simulink model "Model_HVAC_old_controller"  (R2019b)
settings: Solver=VariableStepAuto  StartTime=0.0  StopTime=365*24  RelTol=1e-3
undefined symbols (not defined in the file or in its folder): sigbuilder_block, T_s_in
libraries: simulink x1
(part 1 of 2)
settings Model: Creator=HP  LastModifiedBy=HP
settings DebuggingCC: ArithmeticOperatorsInVariantConditions=warning
settings SFSimCC: CustomCodeUndefinedFunction=UseInterfaceOnly

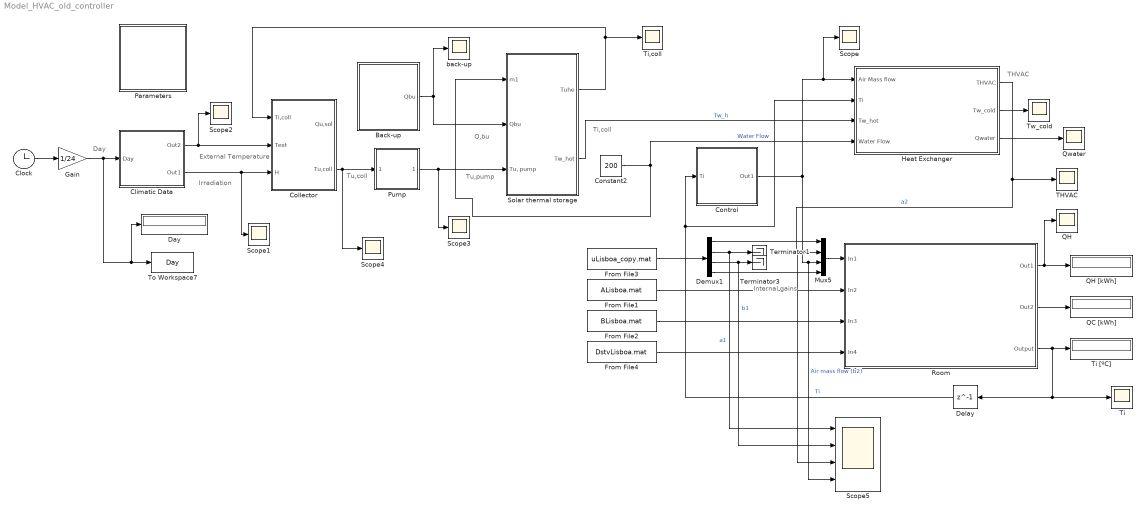
== system Model_HVAC_old_controller ==
  note: THVAC
  note: Internal gains
  note: Tu,pump
  note: Tu,coll
  note: Q,bu
  note: Irradiation
  note: Day
  note: External Temperature
  note: Ti,coll
  Back-up : Subsystem
      mask Display: image(imread('caldaia.jpg'))
  Climatic Data : Subsystem
      mask Display: image(imread('sole.jpg'))
  Clock : Clock
  Collector : Subsystem
      mask Display: image(imread('collettore.jpg'))
  Constant2 : Constant  Value=200
  Control : Subsystem
      mask Display: image('PID.jpg'); % Use "Edit Image" on toolstrip to change.
  Day : Display
  Delay : Delay  DelayLength=1
  Demux1 : Demux  Outputs=[1 1 1 2]
  From File1 : FromFile  FileName=ALisboa.mat  SampleTime=1
  From File2 : FromFile  FileName=BLisboa.mat  SampleTime=1
  From File3 : FromFile  FileName=uLisboa_copy.mat  SampleTime=1
  From File4 : FromFile  FileName=DstvLisboa.mat  SampleTime=1
  Gain : Gain  Gain=1/24  SaturateOnIntegerOverflow=on  OutDataTypeStr=Inherit: Same as input  ParamDataTypeStr=Inherit: Same as input
  Heat Exchanger : Subsystem
      mask Display: image('HE2.jpg'); % Use "Edit Image" on toolstrip to change.
  Mux5 : Mux
  Parameters : Subsystem  mask{Gamma=0, Rho=0.2, Lat=38.74, Beta=45, Eta0=0.959, a1=8.91, a2=0.047, Nc=1, Aap=2.31, m_brine=0.010, Cp_brine=3900, L=1.7, Eta_pump=0.8, Eta_el=0.95, H_pressure=50000, Pump_power=65, Rho_brine=1037, T_room=20, BU_power=2000, Rho_water=1000, Cp_water=4186, U_s=1, T_s_in=45, D_s=0.6, V_s=168, H_s=0.99, UA_s_ex=167, T_s_max=90, A_s_ex=1.8, U_s_ex=1.1, T_DHW=60, S_u=200, T_acq=15}
      mask prompts: Gamma "Azimuth (°)"; Rho "Albedo"; Lat "Latitude (°)"; Beta "Tilt (°)"; Eta0 "Optical efficiency"; a1 "First order coefficient"; a2 "Second order coefficient"; Nc "Number of collectors"; Aap "Absorber area (m2)"; m_brine "Flow rate per surface area (kg/s*m2)"; Cp_brine "Cp brine (J/kgK)"; L "Collector liquid volume (lt)"; Eta_pump "Pump efficiency"; Eta_el "Electrical efficiency"; H_pressure "Head pressure (Pa)"; Pump_power "Pump power (W)"; Rho_brine "Brine density (kg/m3)"; T_room "Room temperature (°C)"; BU_power "Back-up power (W)"; Rho_water "Water density (kg/m3)"; Cp_water "Cp water (J/kgK)"; U_s "Storage U (W/m2K)"; T_s_in "Initial storage temperature (°C)"; D_s "Storage diameter (m)"; V_s "Storage volume (lt)"; H_s "Storage height (m)"; UA_s_ex "Solar exchanger UA (W/K)"; T_s_max "Maximum storage temperature (°C)"; A_s_ex "Heat exchanger area (m2)"; U_s_ex "U-value heat exchanger (W/m2K)"; T_DHW "DHW temperature (°C)"; S_u "Building energetic surface (m2)"; T_acq "Aqueduct temperature (°C)"
      mask Display: image(imread('images.jpg'))
  Pump : Subsystem
      mask Display: image(imread('pompa.jpg'))
  QC [kWh] : Display
      settings: Format=bank  SampleTime=1
  QH : Scope
  QH [kWh] : Display
      settings: Format=bank  SampleTime=1
  Qwater : Scope
  Room : Subsystem
      mask Display: image('roomoffice.jpg'); % Use "Edit Image" on toolstrip to change.
  Scope{,1..4} (5 alike) : Scope
  Scope5 : Scope  NumInputPorts=4
  Solar thermal storage : Subsystem
      mask Display: image(imread('prova.jpg'))
  THVAC : Scope
  Terminator1 : Terminator
  Terminator3 : Terminator
  Ti : Scope
  Ti [ºC] : Display
      settings: Format=bank  SampleTime=1
  Ti,coll : Scope
  To Workspace7 : ToWorkspace  VariableName=Day  SampleTime=[24 0]
  Tw_cold : Scope
  back-up : Scope
  wires:
  Back-up/1(Qbu) -> back-up/1, Solar thermal storage/2(Qbu)
  Solar thermal storage/1(Tuhe) -> Collector/1(Ti,coll), Ti,coll/1
  Gain/1 -> Climatic Data/1(Day), To Workspace7/1, Day/1
  Pump/1(Tu,pump) -> Solar thermal storage/3("Tu, pump"), Scope3/1
  Climatic Data/2(Out1) -> Scope1/1, Collector/3(H)
  Collector/2(Tu,coll) -> Scope4/1, Pump/1(Tu,coll)
  Climatic Data/1(Out2) -> Collector/2(Text), Scope2/1
  Clock/1 -> Gain/1
  Solar thermal storage/2(Tw_hot) -> Heat Exchanger/3(Tw_hot)  "Tw_h"
  Control/1(Out1) -> Scope5/4, Mux5/3, Scope/1, Heat Exchanger/1(Air Mass flow)  "Air mass flow (b2)"
  Heat Exchanger/1(THVAC) -> Scope5/3, Mux5/2, THVAC/1  "a2"
  Heat Exchanger/3(Qwater) -> Qwater/1
  Mux5/1 -> Room/1(In1)
  Heat Exchanger/2(Tw_cold) -> Tw_cold/1
  Delay/1 -> Heat Exchanger/2(Ti), Control/1("Ti ")  "Ti"
  Constant2/1 -> Heat Exchanger/4(Water Flow), Solar thermal storage/1(m1)  "Water Flow"
  Room/3(Output) -> Ti [ºC]/1, Delay/1, Ti/1
  Demux1/3 -> Scope5/2, Terminator3/1  "b1"
  From File4/1 -> Room/4(In4)
  Demux1/2 -> Scope5/1, Terminator1/1  "a1"
  Room/1(Out1) -> QH/1, QH [kWh]/1
  Demux1/4 -> Mux5/4
  From File1/1 -> Room/2(In2)
  From File2/1 -> Room/3(In3)
  Room/2(Out2) -> QC [kWh]/1
  Demux1/1 -> Mux5/1
  From File3/1 -> Demux1/1

== system Model_HVAC_old_controller/Back-up ==
  -Scope : Scope
  -Scope2 : Scope
  Add1 : Sum  Inputs=-+
  Back-up energy [MJ] : Display
  Back-up energy [kWh] : Display
  Constant : Constant  Value=60
  Integral Block : Subsystem
  Product3 : Product  Inputs=**  SaturateOnIntegerOverflow=on  OutDataTypeStr=Inherit: Same as first input
  Prova back-up : Subsystem
  Relay : Relay  OnSwitchValue=0  OffSwitchValue=-5
  Scope : Scope
  To Workspace1 : ToWorkspace  VariableName=Ebu  SampleTime=-1
  To Workspace6 : ToWorkspace  VariableName=Qbu  SampleTime=-1
  Qbu : Outport
  tag scope: Qbu=global
  wires:
  [T3] -> -Scope/1, Add1/1
  Add1/1 -> Relay/1, -Scope2/1
  Relay/1 -> Product3/2
  [BU_power] -> Product3/1
  Product3/1 -> Integral Block/1(Watt), [Qbu], To Workspace6/1, Qbu/1, Scope/1
  Integral Block/1(MJ) -> Back-up energy [MJ]/1
  Integral Block/2(kWh) -> Back-up energy [kWh]/1, To Workspace1/1
  [Tw_hot] -> Add1/2  "Tw_h"
  Constant/1 -> [Tw_hot]

== system Model_HVAC_old_controller/Climatic Data ==
  Day : Inport
  Day Length [h] : Display
  Irradiation : Subsystem  Tag=STV Subsys  LoadFcn=sigbuilder_block('load');  StartFcn=sigbuilder_block('start');  StopFcn=sigbuilder_block('stop');  ClipboardFcn=sigbuilder_block('clipboard');  mask(Sigbuilder block){tuvar=[0:10]}
      mask help: Simulink:masks:SigbuilderBlock_MD
      mask init:
      | if ~strcmp(get_param(bdroot(gcbh),'SimulationStatus'),'stopped') tuvar = sigbuilder_block('maskInit'); end
      settings: CopyFcn=sigbuilder_block('copy');  DeleteFcn=sigbuilder_block('delete');  ModelCloseFcn=sigbuilder_block('modelClose');  PreSaveFcn=sigbuilder_block('preSave');  PauseFcn=sigbuilder_block('pause');  ContinueFcn=sigbuilder_block('continue');  NameChangeFcn=sigbuilder_block('namechange');  OpenFcn=sigbuilder_block('open',[252.75 128.25 550.5 359.25 ]);  CloseFcn=sigbuilder_block('close');
      mask Display: plot(0, 0, 100, 100,[2, 2, 32, 32, 2], [68, 8, 8, 68, 68],[32, 2], [38, 38], [32, 19, 2],[53, 60, 44], [32, 17, 17, 2],[16, 16, 31, 31]);txt = getActiveGroup(gcbh);text(2, 100, txt,'verticalAlignment', 'top');
  Mux4 : Mux  Inputs=2
  Scope : Scope
  Scope1 : Scope
  Scope16 : Scope
  Signal Builder1 : Subsystem  Tag=STV Subsys  LoadFcn=sigbuilder_block('load');  StartFcn=sigbuilder_block('start');  StopFcn=sigbuilder_block('stop');  ClipboardFcn=sigbuilder_block('clipboard');  mask(Sigbuilder block){tuvar=[0:10]}
      mask help: Simulink:masks:SigbuilderBlock_MD
      mask init:
      | if ~strcmp(get_param(bdroot(gcbh),'SimulationStatus'),'stopped') tuvar = sigbuilder_block('maskInit'); end
      settings: CopyFcn=sigbuilder_block('copy');  DeleteFcn=sigbuilder_block('delete');  ModelCloseFcn=sigbuilder_block('modelClose');  PreSaveFcn=sigbuilder_block('preSave');  PauseFcn=sigbuilder_block('pause');  ContinueFcn=sigbuilder_block('continue');  NameChangeFcn=sigbuilder_block('namechange');  OpenFcn=sigbuilder_block('open',[437.6 153 550.4 359.25 ]);  CloseFcn=sigbuilder_block('close');
      mask Display: plot(0, 0, 100, 100,[2, 2, 32, 32, 2], [68, 8, 8, 68, 68],[32, 2], [38, 38], [32, 19, 2],[53, 60, 44], [32, 17, 17, 2],[16, 16, 31, 31]);txt = getActiveGroup(gcbh);text(2, 100, txt,'verticalAlignment', 'top');
  Signal Builder2 : Subsystem  Tag=STV Subsys  LoadFcn=sigbuilder_block('load');  StartFcn=sigbuilder_block('start');  StopFcn=sigbuilder_block('stop');  ClipboardFcn=sigbuilder_block('clipboard');  mask(Sigbuilder block){tuvar=[0:10]}
      mask help: Simulink:masks:SigbuilderBlock_MD
      mask init:
      | if ~strcmp(get_param(bdroot(gcbh),'SimulationStatus'),'stopped') tuvar = sigbuilder_block('maskInit'); end
      settings: CopyFcn=sigbuilder_block('copy');  DeleteFcn=sigbuilder_block('delete');  ModelCloseFcn=sigbuilder_block('modelClose');  PreSaveFcn=sigbuilder_block('preSave');  PauseFcn=sigbuilder_block('pause');  ContinueFcn=sigbuilder_block('continue');  NameChangeFcn=sigbuilder_block('namechange');  OpenFcn=sigbuilder_block('open',[426 129 550.5 359.25 ]);  CloseFcn=sigbuilder_block('close');
      mask Display: plot(0, 0, 100, 100,[2, 2, 32, 32, 2], [68, 8, 8, 68, 68],[32, 2], [38, 38], [32, 19, 2],[53, 60, 44], [32, 17, 17, 2],[16, 16, 31, 31]);txt = getActiveGroup(gcbh);text(2, 100, txt,'verticalAlignment', 'top');
  Signal Builder3 : Subsystem  Tag=STV Subsys  LoadFcn=sigbuilder_block('load');  StartFcn=sigbuilder_block('start');  StopFcn=sigbuilder_block('stop');  ClipboardFcn=sigbuilder_block('clipboard');  mask(Sigbuilder block){tuvar=[0:10]}
      mask help: Simulink:masks:SigbuilderBlock_MD
      mask init:
      | if ~strcmp(get_param(bdroot(gcbh),'SimulationStatus'),'stopped') tuvar = sigbuilder_block('maskInit'); end
      settings: CopyFcn=sigbuilder_block('copy');  DeleteFcn=sigbuilder_block('delete');  ModelCloseFcn=sigbuilder_block('modelClose');  PreSaveFcn=sigbuilder_block('preSave');  PauseFcn=sigbuilder_block('pause');  ContinueFcn=sigbuilder_block('continue');  NameChangeFcn=sigbuilder_block('namechange');  OpenFcn=sigbuilder_block('open',[0 30 1024.5 488.25 ]);  CloseFcn=sigbuilder_block('close');
      mask Display: plot(0, 0, 100, 100,[2, 2, 32, 32, 2], [68, 8, 8, 68, 68],[32, 2], [38, 38], [32, 19, 2],[53, 60, 44], [32, 17, 17, 2],[16, 16, 31, 31]);txt = getActiveGroup(gcbh);text(2, 100, txt,'verticalAlignment', 'top');
  Signal Builder4 : Subsystem  Tag=STV Subsys  LoadFcn=sigbuilder_block('load');  StartFcn=sigbuilder_block('start');  StopFcn=sigbuilder_block('stop');  ClipboardFcn=sigbuilder_block('clipboard');  mask(Sigbuilder block){tuvar=[0:10]}
      mask help: Simulink:masks:SigbuilderBlock_MD
      mask init:
      | if ~strcmp(get_param(bdroot(gcbh),'SimulationStatus'),'stopped') tuvar = sigbuilder_block('maskInit'); end
      settings: CopyFcn=sigbuilder_block('copy');  DeleteFcn=sigbuilder_block('delete');  ModelCloseFcn=sigbuilder_block('modelClose');  PreSaveFcn=sigbuilder_block('preSave');  PauseFcn=sigbuilder_block('pause');  ContinueFcn=sigbuilder_block('continue');  NameChangeFcn=sigbuilder_block('namechange');  OpenFcn=sigbuilder_block('open',[437.6 153 550.4 359.25 ]);  CloseFcn=sigbuilder_block('close');
      mask Display: plot(0, 0, 100, 100,[2, 2, 32, 32, 2], [68, 8, 8, 68, 68],[32, 2], [38, 38], [32, 19, 2],[53, 60, 44], [32, 17, 17, 2],[16, 16, 31, 31]);txt = getActiveGroup(gcbh);text(2, 100, txt,'verticalAlignment', 'top');
  Signal Builder5 : Subsystem  Tag=STV Subsys  LoadFcn=sigbuilder_block('load');  StartFcn=sigbuilder_block('start');  StopFcn=sigbuilder_block('stop');  ClipboardFcn=sigbuilder_block('clipboard');  mask(Sigbuilder block){tuvar=[0:10]}
      mask help: Simulink:masks:SigbuilderBlock_MD
      mask init:
      | if ~strcmp(get_param(bdroot(gcbh),'SimulationStatus'),'stopped') tuvar = sigbuilder_block('maskInit'); end
      settings: CopyFcn=sigbuilder_block('copy');  DeleteFcn=sigbuilder_block('delete');  ModelCloseFcn=sigbuilder_block('modelClose');  PreSaveFcn=sigbuilder_block('preSave');  PauseFcn=sigbuilder_block('pause');  ContinueFcn=sigbuilder_block('continue');  NameChangeFcn=sigbuilder_block('namechange');  OpenFcn=sigbuilder_block('open',[437.6 153 550.4 359.25 ]);  CloseFcn=sigbuilder_block('close');
      mask Display: plot(0, 0, 100, 100,[2, 2, 32, 32, 2], [68, 8, 8, 68, 68],[32, 2], [38, 38], [32, 19, 2],[53, 60, 44], [32, 17, 17, 2],[16, 16, 31, 31]);txt = getActiveGroup(gcbh);text(2, 100, txt,'verticalAlignment', 'top');
  To Workspace2 : ToWorkspace  VariableName=Text  SampleTime=[24 0]
  irraggiamento : Subsystem
  Out2 : Outport  VectorParamsAs1DForOutWhenUnconnected=off
  Out1 : Outport  Port=2  VectorParamsAs1DForOutWhenUnconnected=off
  tag scope: H=global
  wires:
  irraggiamento/1(Out1) -> Day Length [h]/1, Out1/1, Scope/1, [H]
  Mux4/1 -> irraggiamento/1(Climatic Data Input)
  Day/1 -> Mux4/1
  Signal Builder1/1(Temperature) -> Scope16/1, To Workspace2/1, Out2/1
  Irradiation/1(W_45) -> Mux4/2, Scope1/1

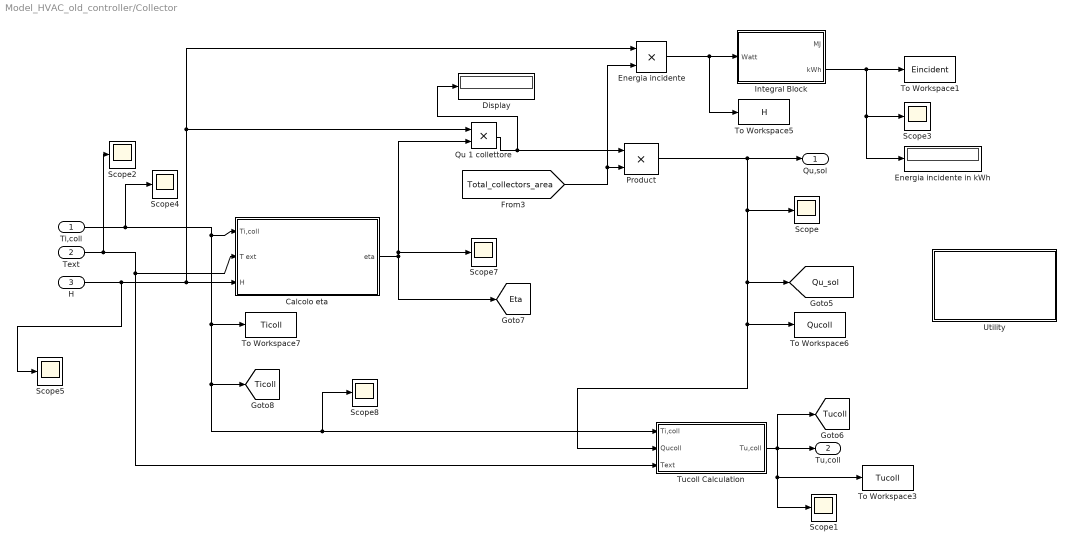
== system Model_HVAC_old_controller/Collector ==
  Ti,coll : Inport
  Text : Inport  Port=2
  H : Inport  Port=3
  Calcolo eta : Subsystem
  Display : Display
  Energia incidente : Product  RndMeth=Zero
  Energia incidente in kWh : Display
  Integral Block : Subsystem
  Product : Product  RndMeth=Zero
  Qu 1 collettore : Product  RndMeth=Zero
  Scope{,1..5,7..8} (8 alike) : Scope
  To Workspace1 : ToWorkspace  VariableName=Eincident  SampleTime=[24 0]
  To Workspace3 : ToWorkspace  VariableName=Tucoll  SampleTime=[24 0]
  To Workspace5 : ToWorkspace  VariableName=H  SampleTime=-1
  To Workspace6 : ToWorkspace  VariableName=Qucoll  SampleTime=[24 0]
  To Workspace7 : ToWorkspace  VariableName=Ticoll  SampleTime=[24 0]
  Tucoll Calculation : Subsystem
  Utility : Subsystem
  Qu,sol : Outport  VectorParamsAs1DForOutWhenUnconnected=off
  Tu,coll : Outport  Port=2  VectorParamsAs1DForOutWhenUnconnected=off
  tag scope: Eta=global, Qu_sol=global, Ticoll=global, Tucoll=global
  wires:
  H/1 -> Scope5/1, Calcolo eta/3(H), Qu 1 collettore/1, Energia incidente/1
  Text/1 -> Scope2/1, Calcolo eta/2(T ext), Tucoll Calculation/3(Text)
  Calcolo eta/1(eta) -> Qu 1 collettore/2, Scope7/1, [Eta]
  Qu 1 collettore/1 -> Product/1, Display/1
  Tucoll Calculation/1(Tu,coll) -> Tu,coll/1, Scope1/1, To Workspace3/1, [Tucoll]
  Energia incidente/1 -> Integral Block/1(Watt), To Workspace5/1
  Product/1 -> Qu,sol/1, [Qu_sol], To Workspace6/1, Tucoll Calculation/2(Qucoll), Scope/1
  Ti,coll/1 -> Scope4/1, [Ticoll], Tucoll Calculation/1(Ti,coll), Scope8/1, To Workspace7/1, Calcolo eta/1(Ti,coll)
  Integral Block/2(kWh) -> To Workspace1/1, Scope3/1, Energia incidente in kWh/1
  [Total_collectors_area] -> Product/2, Energia incidente/2

== system Model_HVAC_old_controller/Control ==
  "Ti " : Inport
  Constant : Constant  Value=24
  Discrete PID Controller (2DOF)1 : simulink/Continuous/PID Controller (2DOF)  Controller=PID  Form=Parallel  TimeDomain=Discrete-time  SampleTime=-1  IntegratorMethod=Forward Euler  FilterMethod=Forward Euler  ControllerParametersSource=internal  P=500  I=100  D=0  UseFilter=on  N=100  b=1  c=1  TunerSelectOption=Transfer Function Based (PID Tuner App)  InitialConditionSource=internal  InitialConditionForIntegrator=0  InitialConditionForFilter=0  DifferentiatorICPrevScaledInput=0  ExternalReset=none  TrackingMode=off  Kt=1  LimitOutput=off  UpperSaturationLimit=inf  LowerSaturationLimit=-inf  LinearizeAsGain=off  AntiWindupMode=none  Kb=1  POutMin=[]  POutMax=[]  IOutMin=[]  IOutMax=[]  DOutMin=[]  DOutMax=[]  NOutMin=[]  NOutMax=[]  bOutMin=[]  bOutMax=[]  cOutMin=[]  cOutMax=[]  SumOutMin=[]  SumOutMax=[]  SaturationOutMin=[]  SaturationOutMax=[]  PParamMin=[]  PParamMax=[]  IParamMin=[]  IParamMax=[]  DParamMin=[]  DParamMax=[]  NParamMin=[]  NParamMax=[]  bParamMin=[]  bParamMax=[]  cParamMin=[]  cParamMax=[]  KbParamMin=[]  KbParamMax=[]  KtParamMin=[]  KtParamMax=[]  KbOutMin=[]  KbOutMax=[]  KtOutMin=[]  KtOutMax=[]  IntegratorOutMin=[]  IntegratorOutMax=[]  FilterOutMin=[]  FilterOutMax=[]  SumI1OutMin=[]  SumI1OutMax=[]  SumI2OutMin=[]  SumI2OutMax=[]  SumI3OutMin=[]  SumI3OutMax=[]  SumI4OutMin=[]  SumI4OutMax=[]  SumDOutMin=[]  SumDOutMax=[]  Sum1OutMin=[]  Sum1OutMax=[]  Sum2OutMin=[]  Sum2OutMax=[]  Sum3OutMin=[]  Sum3OutMax=[]  DifferentiatorOutMin=[]  DifferentiatorOutMax=[]  FilterDiffOutCoefMin=[]  FilterDiffOutCoefMax=[]  ReciprocalOutMin=[]  ReciprocalOutMax=[]  SumDenOutMin=[]  SumDenOutMax=[]  SumNumOutMin=[]  SumNumOutMax=[]  DivideOutMin=[]  DivideOutMax=[]  IntegratorContinuousStateAttributes=''  IntegratorStateMustResolveToSignalObject=off  IntegratorRTWStateStorageClass=Auto  FilterContinuousStateAttributes=''  FilterStateMustResolveToSignalObject=off  FilterRTWStateStorageClass=Auto  ParallelPVariant=InternalParameters  IdealPVariant=Disabled  IVariant=InternalParameters  DVariant=InternalParameters  bVariant=InternalParameters  cVariant=InternalParameters  IntegratorVariant=Discrete  SatVariant=Disabled  AWVariant=Passthrough  PCopyVariant=Disabled  TRVariant=Disabled  FdbkBlocksVariant=Forward  IdealPFdbkVariant=Disabled  SatFdbkVariant=Disabled  DerivativeFilterVariant=ForwardEulerFilter  NVariant=InternalParameters  NCopyVariant=Disabled  FilterICVariant=InternalICsFilter  IntegratorICVariant=InternalICs  ExternalResetVariant=Disabled  TRSumVariant=Passthrough  SumFdbkVariant=Disabled  SumVariant=Sum_PID
  Saturation : Saturate  UpperLimit=1000  LowerLimit=0
  Scope3 : Scope
  Out1 : Outport
  wires:
  Saturation/1 -> Out1/1, Scope3/1  "Air mass flow"
  Discrete PID Controller (2DOF)1/1 -> Saturation/1  "Air mass flow"
  Constant/1 -> Discrete PID Controller (2DOF)1/1
  "Ti "/1 -> Discrete PID Controller (2DOF)1/2

== system Model_HVAC_old_controller/Heat Exchanger ==
  Air Mass flow : Inport
  Ti : Inport  Port=2
  Tw_hot : Inport  Port=3
  Water Flow : Inport  Port=4
  Add : Sum
  Add1 : Sum  Inputs=+-
  Add2 : Sum  Inputs=+-
  Cpair : Constant  Value=1.007
  Cpwater : Constant  Value=4.17
  Divide : Product  Inputs=/**
  Divide1 : Product  Inputs=***
  Divide3 : Product  Inputs=/**
  efficiency : Constant  Value=0.7
  THVAC : Outport
  Tw_cold : Outport  Port=2
  Qwater : Outport  Port=3
  wires:
  Cpair/1 -> Divide1/3, Divide/3
  Air Mass flow/1 -> Divide/2
  Divide/1 -> Add/1
  Ti/1 -> Add/2, Add1/2
  Add/1 -> THVAC/1
  efficiency/1 -> Divide1/2
  Tw_hot/1 -> Add2/1, Add1/1
  Add1/1 -> Divide1/1
  Divide1/1 -> Qwater/1, Divide3/1, Divide/1
  Water Flow/1 -> Divide3/2
  Cpwater/1 -> Divide3/3
  Divide3/1 -> Add2/2
  Add2/1 -> Tw_cold/1

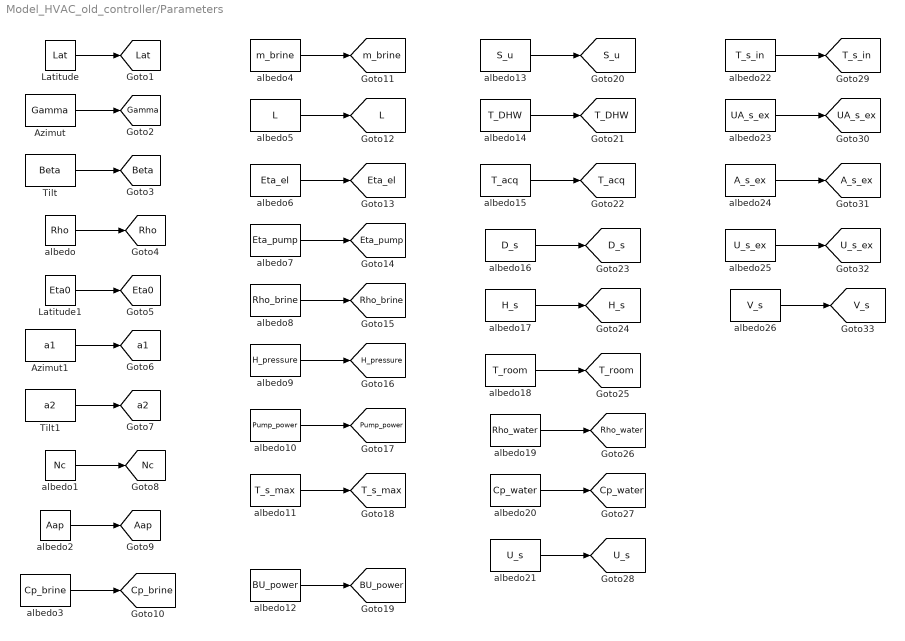
== system Model_HVAC_old_controller/Parameters ==
  Azimut : Constant  Value=Gamma
  Azimut1 : Constant  Value=a1
  Latitude : Constant  Value=Lat
  Latitude1 : Constant  Value=Eta0
  Tilt : Constant  Value=Beta
  Tilt1 : Constant  Value=a2
  albedo : Constant  Value=Rho
  albedo1 : Constant  Value=Nc
  albedo10 : Constant  Value=Pump_power
  albedo11 : Constant  Value=T_s_max
  albedo12 : Constant  Value=BU_power
  albedo13 : Constant  Value=S_u
  albedo14 : Constant  Value=T_DHW
  albedo15 : Constant  Value=T_acq
  albedo16 : Constant  Value=D_s
  albedo17 : Constant  Value=H_s
  albedo18 : Constant  Value=T_room
  albedo19 : Constant  Value=Rho_water
  albedo2 : Constant  Value=Aap
  albedo20 : Constant  Value=Cp_water
  albedo21 : Constant  Value=U_s
  albedo22 : Constant  Value=T_s_in
  albedo23 : Constant  Value=UA_s_ex
  albedo24 : Constant  Value=A_s_ex
  albedo25 : Constant  Value=U_s_ex
  albedo26 : Constant  Value=V_s
  albedo3 : Constant  Value=Cp_brine
  albedo4 : Constant  Value=m_brine
  albedo5 : Constant  Value=L
  albedo6 : Constant  Value=Eta_el
  albedo7 : Constant  Value=Eta_pump
  albedo8 : Constant  Value=Rho_brine
  albedo9 : Constant  Value=H_pressure
  tag scope: A_s_ex=global, Aap=global, BU_power=global, Beta=global, Cp_brine=global, Cp_water=global, D_s=global, Eta0=global, Eta_el=global, Eta_pump=global, Gamma=global, H_pressure=global, H_s=global, L=global, Lat=global, Nc=global, Pump_power=global, Rho=global, Rho_brine=global, Rho_water=global, S_u=global, T_DHW=global, T_acq=global, T_room=global, T_s_in=global, T_s_max=global, UA_s_ex=global, U_s=global, U_s_ex=global, V_s=global, a1=global, a2=global, m_brine=global
  wires:
  Latitude/1 -> [Lat]
  Azimut/1 -> [Gamma]
  Tilt/1 -> [Beta]
  albedo/1 -> [Rho]
  Latitude1/1 -> [Eta0]
  Azimut1/1 -> [a1]
  Tilt1/1 -> [a2]
  albedo1/1 -> [Nc]
  albedo2/1 -> [Aap]
  albedo3/1 -> [Cp_brine]
  albedo4/1 -> [m_brine]
  albedo5/1 -> [L]
  albedo6/1 -> [Eta_el]
  albedo7/1 -> [Eta_pump]
  albedo8/1 -> [Rho_brine]
  albedo9/1 -> [H_pressure]
  albedo10/1 -> [Pump_power]
  albedo11/1 -> [T_s_max]
  albedo12/1 -> [BU_power]
  albedo13/1 -> [S_u]
  albedo14/1 -> [T_DHW]
  albedo15/1 -> [T_acq]
  albedo16/1 -> [D_s]
  albedo17/1 -> [H_s]
  albedo18/1 -> [T_room]
  albedo19/1 -> [Rho_water]
  albedo20/1 -> [Cp_water]
  albedo21/1 -> [U_s]
  albedo22/1 -> [T_s_in]
  albedo23/1 -> [UA_s_ex]
  albedo24/1 -> [A_s_ex]
  albedo25/1 -> [U_s_ex]
  albedo26/1 -> [V_s]

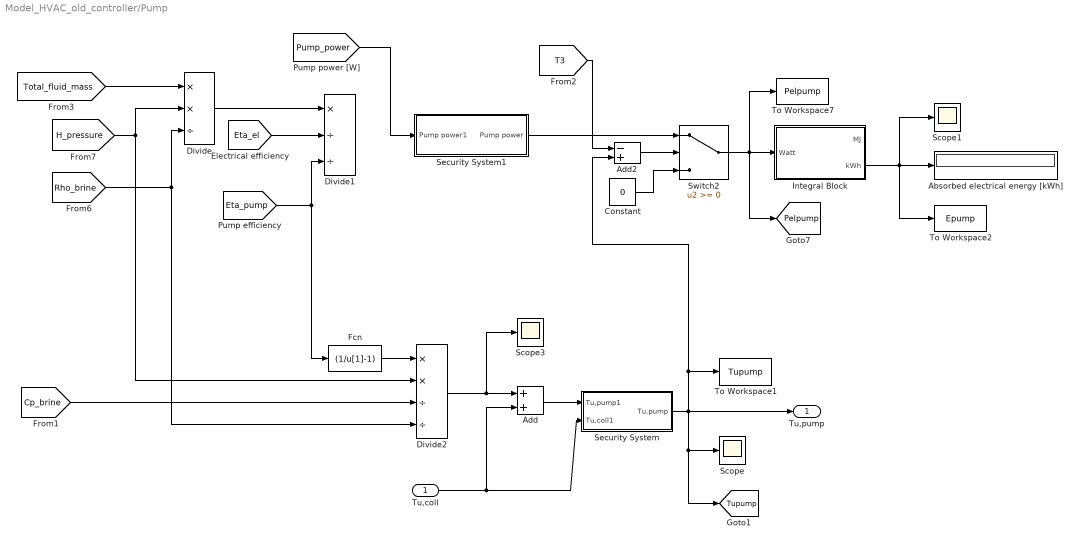
== system Model_HVAC_old_controller/Pump ==
  Tu,coll : Inport
  Absorbed electrical energy [kWh] : Display
  Add : Sum
  Add2 : Sum  Inputs=-+
  Constant : Constant  Value=0
  Divide : Product  Inputs=**/
  Divide1 : Product  Inputs=*//
  Divide2 : Product  Inputs=**//
  Fcn : Fcn  Expr=(1/u[1]-1)
  Integral Block : Subsystem
  Scope : Scope
  Scope1 : Scope
  Scope3 : Scope
  Security System : Subsystem
  Security System1 : Subsystem
  Switch2 : Switch  ZeroCross=off
  To Workspace1 : ToWorkspace  VariableName=Tupump  SampleTime=[24 0]
  To Workspace2 : ToWorkspace  VariableName=Epump  SampleTime=[24 0]
  To Workspace7 : ToWorkspace  VariableName=Pelpump  SampleTime=[24 0]
  Tu,pump : Outport  VectorParamsAs1DForOutWhenUnconnected=off
  tag scope: Pelpump=global, Tupump=global
  wires:
  [Total_fluid_mass] -> Divide/1
  [H_pressure] -> Divide/2, Divide2/2
  [Rho_brine] -> Divide/3, Divide2/4
  Divide/1 -> Divide1/1
  [Eta_pump] -> Fcn/1, Divide1/3
  Fcn/1 -> Divide2/1
  Divide2/1 -> Add/1, Scope3/1
  Tu,coll/1 -> Security System/2(Tu,coll1), Add/2
  [Cp_brine] -> Divide2/3
  Integral Block/2(kWh) -> Absorbed electrical energy [kWh]/1, Scope1/1, To Workspace2/1
  Add/1 -> Security System/1(Tu,pump1)
  Security System/1(Tu,pump) -> To Workspace1/1, Add2/2, Scope/1, [Tupump], Tu,pump/1
  [Eta_el] -> Divide1/2
  [Pump_power] -> Security System1/1(Pump power1)
  Security System1/1(Pump power) -> Switch2/1
  Add2/1 -> Switch2/2
  [T3] -> Add2/1
  Switch2/1 -> To Workspace7/1, [Pelpump], Integral Block/1(Watt)
  Constant/1 -> Switch2/3

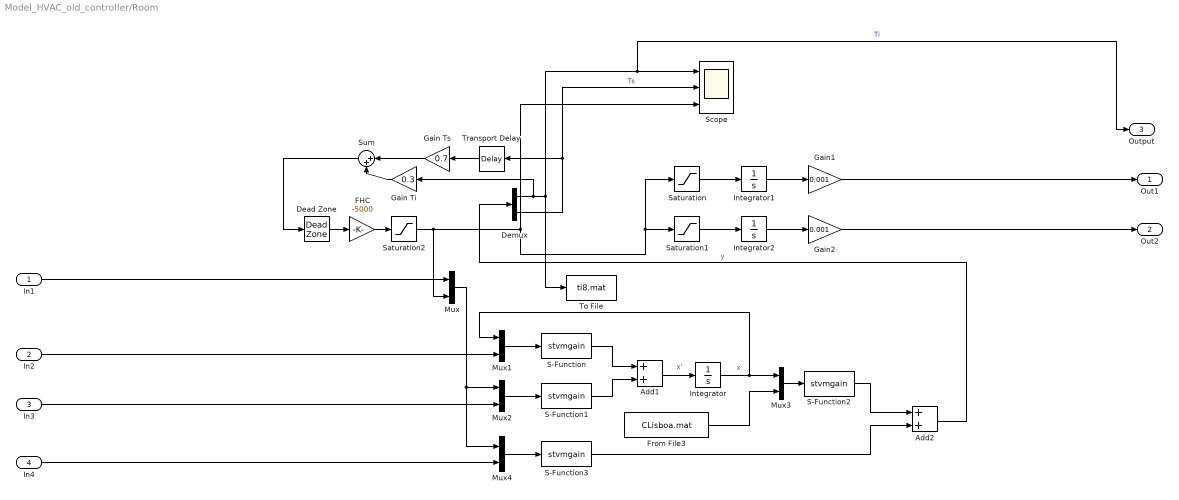
== system Model_HVAC_old_controller/Room ==
  note: x'
  note: x
  In1 : Inport
  In2 : Inport  Port=2
  In3 : Inport  Port=3
  In4 : Inport  Port=4
  Add1 : Sum
  Add2 : Sum
  Dead Zone : DeadZone  LowerValue=20  UpperValue=26  ZeroCross=off  SaturateOnIntegerOverflow=on
  Demux : Demux  Outputs=2
  FHC : Gain  Gain=-5000
  From File3 : FromFile  FileName=CLisboa.mat  SampleTime=1
  Gain Ti : Gain  Gain=0.3
  Gain Ts : Gain  Gain=0.7
  Gain1 : Gain  Gain=0.001  SampleTime=1
  Gain2 : Gain  Gain=0.001  SampleTime=1
  Integrator : Integrator  InitialCondition=18
  Integrator1 : Integrator
  Integrator2 : Integrator
  Mux : Mux  Inputs=2
  Mux1 : Mux  Inputs=[1 1]
  Mux2 : Mux  Inputs=[6 6]
  Mux3 : Mux  Inputs=[1 2]
  Mux4 : Mux  Inputs=[6 12]
  S-Function : S-Function  FunctionName=stvmgain  Parameters=1, -1  SFunctionDeploymentMode=off  EnableBusSupport=off
  S-Function1 : S-Function  FunctionName=stvmgain  Parameters=[1 1 1 1 1 1], -1  SFunctionDeploymentMode=off  EnableBusSupport=off
  S-Function2 : S-Function  FunctionName=stvmgain  Parameters=[1 ;1] -1  SFunctionDeploymentMode=off  EnableBusSupport=off
  S-Function3 : S-Function  FunctionName=stvmgain  Parameters=[1 1 1 1 1 1; 1 1 1 1 1 1], -1  SFunctionDeploymentMode=off  EnableBusSupport=off
  Saturation : Saturate  UpperLimit=20000  LowerLimit=0  SampleTime=1
  Saturation1 : Saturate  UpperLimit=0  LowerLimit=-20000  SampleTime=1
  Saturation2 : Saturate  UpperLimit=10000  LowerLimit=-10000
  Scope : Scope  NumInputPorts=3
  Sum : Sum  Inputs=|++
  To File : ToFile  Filename=ti8.mat  SampleTime=1
  Transport Delay : TransportDelay
  Out1 : Outport  VectorParamsAs1DForOutWhenUnconnected=off
  Out2 : Outport  Port=2  VectorParamsAs1DForOutWhenUnconnected=off
  Output : Outport  Port=3  VectorParamsAs1DForOutWhenUnconnected=off
  wires:
  Sum/1 -> Dead Zone/1
  Mux3/1 -> S-Function2/1
  Demux/1 -> Gain Ti/1, Output/1, Scope/1, To File/1  "Ti"
  Mux2/1 -> S-Function1/1
  Saturation2/1 -> Mux/2, Scope/3, Saturation1/1, Saturation/1
  Mux/1 -> Mux2/1, Mux4/1
  Saturation/1 -> Integrator1/1
  Gain1/1 -> Out1/1
  S-Function/1 -> Add1/1
  Mux4/1 -> S-Function3/1
  Integrator/1 -> Mux3/1, Mux1/1
  FHC/1 -> Saturation2/1
  Saturation1/1 -> Integrator2/1
  Gain Ts/1 -> Sum/1
  Mux1/1 -> S-Function/1
  S-Function3/1 -> Add2/2
  Transport Delay/1 -> Gain Ts/1
  Dead Zone/1 -> FHC/1
  Gain Ti/1 -> Sum/2
  S-Function1/1 -> Add1/2
  Integrator2/1 -> Gain2/1
  Demux/2 -> Scope/2, Transport Delay/1  "Ts"
  In3/1 -> Mux2/2
  Add1/1 -> Integrator/1
  Gain2/1 -> Out2/1
  From File3/1 -> Mux3/2
  In2/1 -> Mux1/2
  S-Function2/1 -> Add2/1
  Integrator1/1 -> Gain1/1
  Add2/1 -> Demux/1  "y"
  In4/1 -> Mux4/2
  In1/1 -> Mux/1

== system Model_HVAC_old_controller/Solar thermal storage ==
  note: V[m3]
  m1 : Inport
  Qbu : Inport  Port=2
  "Tu, pump" : Inport  Port=3
  -Scope1 : Scope
  Divide : Product  Inputs=*/
  Lower part 3 : Subsystem
  Rho water : Constant  Value=1000
  Scope : Scope
  Scope2 : Scope
  Tuhe : Outport  VectorParamsAs1DForOutWhenUnconnected=off
  Tw_hot : Outport  Port=2
  tag scope: m=global
  wires:
  Divide/1 -> Scope2/1, Lower part 3/1(V)
  Rho water/1 -> Divide/2
  Lower part 3/2(Tuhe) -> Tuhe/1
  "Tu, pump"/1 -> Scope/1, Lower part 3/2(Tupump)
  Qbu/1 -> Lower part 3/3(Qbu), -Scope1/1
  m1/1 -> [m]
  [V_s] -> Divide/1
  Lower part 3/1(Tstorage) -> Tw_hot/1

== system Model_HVAC_old_controller/Back-up/Integral Block ==
  Watt : Inport
  Integrator : Integrator
  J to MJ : Gain  Gain=1/1000000
  MJ to kWh : Gain  Gain=1/3.6
  MJ1 : Display
  Scope1 : Scope
  Scope2 : Scope
  kWh1 : Display
  MJ : Outport  VectorParamsAs1DForOutWhenUnconnected=off
  kWh : Outport  Port=2  VectorParamsAs1DForOutWhenUnconnected=off
  wires:
  Integrator/1 -> J to MJ/1
  Watt/1 -> Integrator/1
  J to MJ/1 -> Scope1/1, MJ1/1, MJ/1, MJ to kWh/1
  MJ to kWh/1 -> Scope2/1, kWh1/1, kWh/1

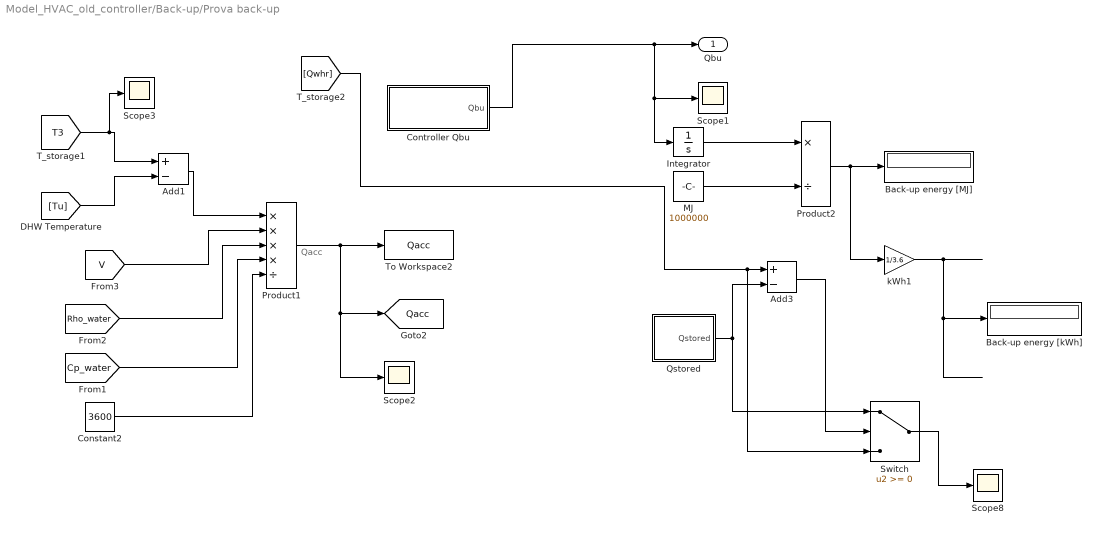
== system Model_HVAC_old_controller/Back-up/Prova back-up ==
  note: Qacc
  Add1 : Sum  Inputs=+-
  Add3 : Sum  Inputs=+-
  Back-up energy [MJ] : Display
  Back-up energy [kWh] : Display
  Constant2 : Constant  Value=3600
  Controller Qbu : Subsystem
  Integrator : Integrator
  MJ : Constant  Value=1000000
  Product1 : Product  Inputs=****/  SaturateOnIntegerOverflow=on  OutDataTypeStr=Inherit: Same as first input
  Product2 : Product  Inputs=*/  SaturateOnIntegerOverflow=on  OutDataTypeStr=Inherit: Same as first input
  Qstored : Subsystem
  Scope{1..3,8} (4 alike) : Scope
  Switch : Switch  ZeroCross=off
  To Workspace2 : ToWorkspace  VariableName=Qacc  SampleTime=[3600 0]
  kWh1 : Gain  Gain=1/3.6
  Qbu : Outport  VectorParamsAs1DForOutWhenUnconnected=off
  tag scope: Qacc=global
  wires:
  [Tu] -> Add1/2
  [T3] -> Add1/1, Scope3/1
  Integrator/1 -> Product2/1
  MJ/1 -> Product2/2
  Product2/1 -> Back-up energy [MJ]/1, kWh1/1
  kWh1/1 -> Back-up energy [kWh]/1
  Add1/1 -> Product1/1
  [V] -> Product1/2
  [Rho_water] -> Product1/3
  Product1/1 -> To Workspace2/1, Scope2/1, [Qacc]
  [Cp_water] -> Product1/4
  Constant2/1 -> Product1/5
  [Qwhr] -> Add3/1, Switch/3
  Controller Qbu/1(Qbu) -> Qbu/1, Scope1/1, Integrator/1
  Switch/1 -> Scope8/1
  Qstored/1(Qstored) -> Add3/2, Switch/1
  Add3/1 -> Switch/2

== system Model_HVAC_old_controller/Climatic Data/Irradiation ==
  Demux : Demux  Tag=STV Demux  Outputs=2
  FromWs : FromWorkspace  Tag=STV FromWs  VariableName=tuvar  SampleTime=0
      SigBuilderData=|
      | common.afterFinalStr = 'Extrapolate'
      | common.sampleTime = 0
      | dataSet.timeRange = [0 8760]
      | dataSet.name = 'Lisbon'
      | sbobj.Groups.Name = 'Lisbon'
      | sbobj.Groups.Signals(1).Name = 'W_45'
      | sbobj.Groups.Signals(1).XData = [0 2 3 4 5 6 7 8 9 10 11 12 ... (8759 elements, 1x8759)]
      | sbobj.Groups.Signals(1).YData = [0 0 0 0 0 0 0 0 0 29.1632292207 68.8820068572 90.3706202093 ... (8759 elements, 1x8759)]
      | sbobj.Groups.Signals(2).Name = 'E_45'
      | sbobj.Groups.Signals(2).XData = [0 2 3 4 5 6 7 8 9 10 11 12 ... (8759 elements, 1x8759)]
      | sbobj.Groups.Signals(2).YData = [0 0 0 0 0 0 0 0 0 141.083006062 202.903847513 454.497491992 ... (8759 elements, 1x8759)]
      | sbobj.Groups.TimeRange = [0 8760]
  W_45 : Outport  Tag=STV Outport
  E_45 : Outport  Tag=STV Outport  Port=2
  wires:
  FromWs/1 -> Demux/1
  Demux/1 -> W_45/1
  Demux/2 -> E_45/1

== system Model_HVAC_old_controller/Climatic Data/Signal Builder1 ==
  Demux : Demux  Tag=STV Demux  Outputs=1
  FromWs : FromWorkspace  Tag=STV FromWs  VariableName=tuvar  SampleTime=0
      SigBuilderData=|
      | common.afterFinalStr = 'Extrapolate'
      | common.sampleTime = 0
      | dataSet.timeRange = [0 8760]
      | dataSet.name = 'Lisbon'
      | sbobj.Groups.Name = 'Lisbon'
      | sbobj.Groups.Signals.Name = 'Temperature'
      | sbobj.Groups.Signals.XData = [0 1 2 3 4 5 6 7 8 9 10 11 ... (8761 elements, 1x8761)]
      | sbobj.Groups.Signals.YData = [10.3 10.3 10.5 10.4 10.4 10.3 10.2 10.1 10 10.2 10.7 11.6 ... (8761 elements, 1x8761)]
      | sbobj.Groups.TimeRange = [0 8760]
  Temperature : Outport  Tag=STV Outport
  wires:
  FromWs/1 -> Demux/1
  Demux/1 -> Temperature/1

== system Model_HVAC_old_controller/Climatic Data/Signal Builder2 ==
  Demux : Demux  Tag=STV Demux  Outputs=2
  FromWs : FromWorkspace  Tag=STV FromWs  VariableName=tuvar  SampleTime=0
      SigBuilderData=|
      | common.afterFinalStr = 'Extrapolate'
      | common.sampleTime = 0
      | dataSet.timeRange = [0 8760]
      | dataSet.name = 'Marseille'
      | sbobj.Groups.Name = 'Marseille'
      | sbobj.Groups.Signals(1).Name = 'W_45'
      | sbobj.Groups.Signals(1).XData = [0 2 3 4 5 6 7 8 9 10 11 12 ... (8759 elements, 1x8759)]
      | sbobj.Groups.Signals(1).YData = [0 0 0 0 0 0 0 0 6.17989898732 47.6735064736 135.109148592 252.985100356 ... (8759 elements, 1x8759)]
      | sbobj.Groups.Signals(2).Name = 'E_45'
      | sbobj.Groups.Signals(2).XData = [0 2 3 4 5 6 7 8 9 10 11 12 ... (8759 elements, 1x8759)]
      | sbobj.Groups.Signals(2).YData = [0 0 0 0 0 0 0 0 6.17989898732 47.6735064736 177.771859905 213.255603873 ... (8759 elements, 1x8759)]
      | sbobj.Groups.TimeRange = [0 8760]
  W_45 : Outport  Tag=STV Outport
  E_45 : Outport  Tag=STV Outport  Port=2
  wires:
  FromWs/1 -> Demux/1
  Demux/1 -> W_45/1
  Demux/2 -> E_45/1

== system Model_HVAC_old_controller/Climatic Data/Signal Builder3 ==
  Demux : Demux  Tag=STV Demux  Outputs=2
  FromWs : FromWorkspace  Tag=STV FromWs  VariableName=tuvar  SampleTime=0
      SigBuilderData=|
      | common.afterFinalStr = 'Extrapolate'
      | common.sampleTime = 0
      | dataSet.timeRange = [0 8760]
      | dataSet.name = 'Madrid'
      | sbobj.Groups.Name = 'Madrid'
      | sbobj.Groups.Signals(1).Name = 'W_45'
      | sbobj.Groups.Signals(1).XData = [0 2 3 4 5 6 7 8 9 10 11 12 ... (8759 elements, 1x8759)]
      | sbobj.Groups.Signals(1).YData = [0 0 0 0 0 0 0 0 13.2426406871 26.542132838 43.295004142 60.0723463924 ... (8759 elements, 1x8759)]
      | sbobj.Groups.Signals(2).Name = 'E_45'
      | sbobj.Groups.Signals(2).XData = [0 2 3 4 5 6 7 8 9 10 11 12 ... (8759 elements, 1x8759)]
      | sbobj.Groups.Signals(2).YData = [0 0 0 0 0 0 0 0 13.2426406871 31.8469083409 45.9080836816 62.4618107621 ... (8759 elements, 1x8759)]
      | sbobj.Groups.TimeRange = [0 8760]
  W_45 : Outport  Tag=STV Outport
  E_45 : Outport  Tag=STV Outport  Port=2
  wires:
  FromWs/1 -> Demux/1
  Demux/1 -> W_45/1
  Demux/2 -> E_45/1

== system Model_HVAC_old_controller/Climatic Data/Signal Builder4 ==
  Demux : Demux  Tag=STV Demux  Outputs=1
  FromWs : FromWorkspace  Tag=STV FromWs  VariableName=tuvar  SampleTime=0
      SigBuilderData=|
      | common.afterFinalStr = 'Extrapolate'
      | common.sampleTime = 0
      | dataSet.timeRange = [0 8760]
      | dataSet.name = 'Madrid'
      | sbobj.Groups.Name = 'Madrid'
      | sbobj.Groups.Signals.Name = 'Temperature'
      | sbobj.Groups.Signals.XData = [0 2 3 4 5 6 7 8 9 10 11 12 ... (8759 elements, 1x8759)]
      | sbobj.Groups.Signals.YData = [4.4 4.4 4.4 3.9 3.9 3.3 3.3 2.8 3.3 3.9 5 6.1 ... (8759 elements, 1x8759)]
      | sbobj.Groups.TimeRange = [0 8760]
  Temperature : Outport  Tag=STV Outport
  wires:
  FromWs/1 -> Demux/1
  Demux/1 -> Temperature/1

== system Model_HVAC_old_controller/Climatic Data/Signal Builder5 ==
  Demux : Demux  Tag=STV Demux  Outputs=1
  FromWs : FromWorkspace  Tag=STV FromWs  VariableName=tuvar  SampleTime=0
      SigBuilderData=|
      | common.afterFinalStr = 'Extrapolate'
      | common.sampleTime = 0
      | dataSet.timeRange = [0 8760]
      | dataSet.name = 'Marseille'
      | sbobj.Groups.Name = 'Marseille'
      | sbobj.Groups.Signals.Name = 'Temperature'
      | sbobj.Groups.Signals.XData = [0 1 2 3 4 5 6 7 8 9 10 11 ... (8761 elements, 1x8761)]
      | sbobj.Groups.Signals.YData = [9.4 9.4 8.9 8.6 8.4 8.3 8.1 6.9 5 6 6.3 7 ... (8761 elements, 1x8761)]
      | sbobj.Groups.TimeRange = [0 8760]
  Temperature : Outport  Tag=STV Outport
  wires:
  FromWs/1 -> Demux/1
  Demux/1 -> Temperature/1

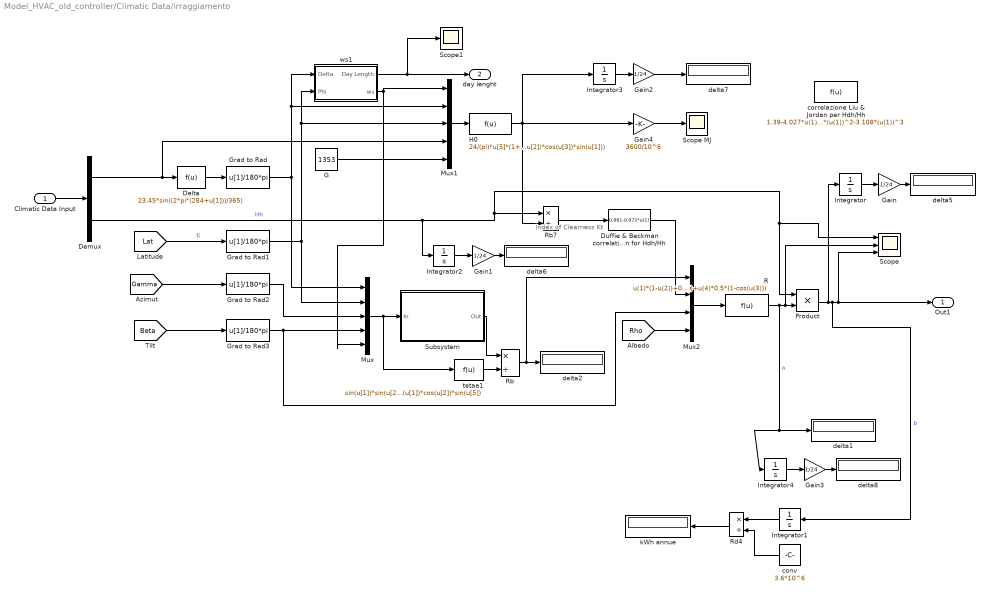
== system Model_HVAC_old_controller/Climatic Data/irraggiamento ==
  note: Index of Clearness Kt
  Climatic Data Input : Inport
  Delta : Fcn  Expr=23.45*sin((2*pi*(284+u[1]))/365)
  Demux : Demux  Outputs=2
  Duffie & Beckman correlation for Hdh/Hh : Fcn  Expr=0.881-0.972*u(1)
  G : Constant  Value=1353
  Gain{,1..3} (4 alike) : Gain  Gain=1/24
  Gain4 : Gain  Gain=3600/10^6
  Grad to Rad{,1..3} (4 alike) : Fcn  Expr=u[1]/180*pi
  H0 : Fcn  Expr=24/(pi)*u[5]*(1+0.033*cos((2*pi*u[4])/365))*(sin(u[2])*sin(u[3])*u(1)+cos(u[2])*cos(u[3])*sin(u[1]))
  Integrator{,1..4} (5 alike) : Integrator
  Mux : Mux  Inputs=5
  Mux1 : Mux  Inputs=5
  Mux2 : Mux
  Product : Product  RndMeth=Zero
  R : Fcn  Expr=u(1)*(1-u(2))+0.5*(1+cos(u(3)))*u(2)+u(4)*0.5*(1-cos(u(3)))
  Rb : Product  Inputs=*/  SaturateOnIntegerOverflow=on  OutDataTypeStr=Inherit: Same as first input
  Rb7 : Product  Inputs=*/  SaturateOnIntegerOverflow=on  OutDataTypeStr=Inherit: Same as first input
  Rd4 : Product  Inputs=*/  SaturateOnIntegerOverflow=on  OutDataTypeStr=Inherit: Same as first input
  Scope : Scope  NumInputPorts=3
  Scope MJ : Scope
  Scope1 : Scope
  Subsystem : Subsystem
  conv : Constant  Value=3.6*10^6
  correlazione Liu & Jordan per Hdh/Hh : Fcn  Expr=1.39-4.027*u(1)+5.531*(u(1))^2-3.108*(u(1))^3
  delta{1..2,5..8} (6 alike) : Display
  kWh annue : Display
  tetaa1 : Fcn  Expr=sin(u[1])*sin(u[2])*u(5)+cos(u[1])*cos(u[2])*sin(u[5])
  ws1 : Subsystem
  Out1 : Outport  VectorParamsAs1DForOutWhenUnconnected=off
  day lenght : Outport  Port=2
  wires:
  Grad to Rad/1 -> ws1/1(Delta), Mux1/2, Mux/1
  Delta/1 -> Grad to Rad/1
  Mux1/1 -> H0/1
  H0/1 -> Integrator3/1, Gain4/1, Rb7/2
  ws1/2(ws) -> Mux1/1, Mux/5
  Climatic Data Input/1 -> Demux/1
  [Lat] -> Grad to Rad1/1  "fi"
  G/1 -> Mux1/5
  Demux/2 -> Integrator2/1, Rb7/1, Scope/1, Product/1  "Hh"
  Rb7/1 -> Duffie & Beckman correlation for Hdh/Hh/1
  Mux/1 -> tetaa1/1, Subsystem/1(In)
  tetaa1/1 -> Rb/2
  Rb/1 -> delta2/1, Mux2/1
  Mux2/1 -> R/1
  [Rho] -> Mux2/4
  Duffie & Beckman correlation for Hdh/Hh/1 -> Mux2/2
  R/1 -> delta1/1, Integrator4/1, Scope/2, Product/2  "a"
  Product/1 -> Scope/3, Out1/1, Integrator1/1, Integrator/1  "b"
  Subsystem/1(Out) -> Rb/1
  Grad to Rad1/1 -> Mux1/3, ws1/2(Phi), Mux/2
  [Gamma] -> Grad to Rad2/1
  Demux/1 -> Delta/1, Mux1/4
  Grad to Rad2/1 -> Mux/3
  [Beta] -> Grad to Rad3/1
  Grad to Rad3/1 -> Mux2/3, Mux/4
  Integrator/1 -> Gain/1
  Gain/1 -> delta5/1
  Integrator1/1 -> Rd4/1
  Rd4/1 -> kWh annue/1
  conv/1 -> Rd4/2
  Integrator2/1 -> Gain1/1
  Gain1/1 -> delta6/1
  Integrator3/1 -> Gain2/1
  Gain2/1 -> delta7/1
  Integrator4/1 -> Gain3/1
  Gain3/1 -> delta8/1
  Gain4/1 -> Scope MJ/1
  ws1/1(Day Length) -> Scope1/1, day lenght/1

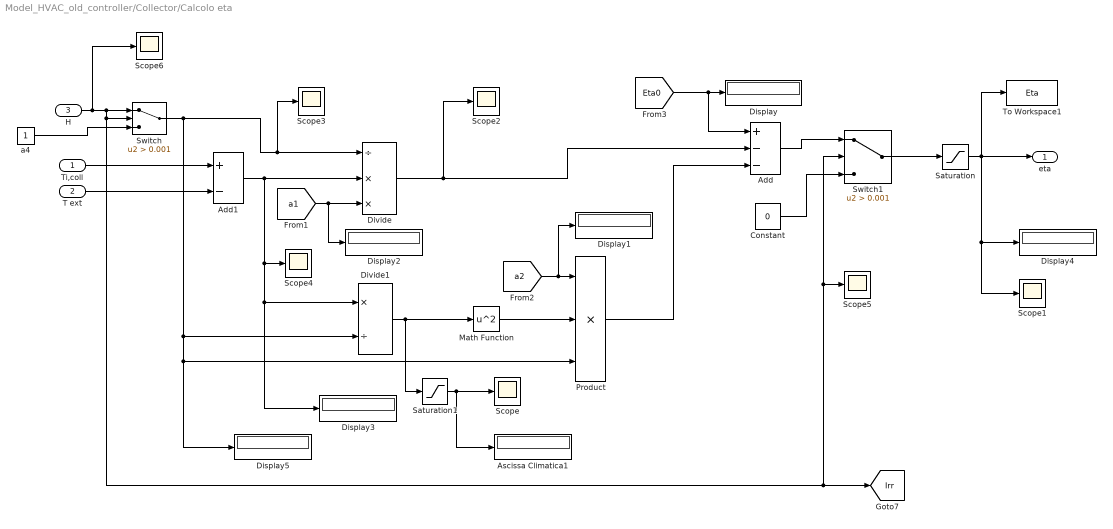
== system Model_HVAC_old_controller/Collector/Calcolo eta ==
  Ti,coll : Inport
  T ext : Inport  Port=2
  H : Inport  Port=3
  Add : Sum  Inputs=+--
  Add1 : Sum  Inputs=+-
  Ascissa Climatica1 : Display
  Constant : Constant  Value=0
  Display{,1..5} (6 alike) : Display
  Divide : Product  Inputs=/**
  Divide1 : Product  Inputs=*/
  Math Function : Math  Operator=square  SaturateOnIntegerOverflow=on
  Product : Product  Inputs=3  RndMeth=Zero
  Saturation : Saturate  UpperLimit=1  LowerLimit=-inf
  Saturation1 : Saturate  UpperLimit=1  LowerLimit=0
  Scope{,1..6} (7 alike) : Scope
  Switch : Switch  Criteria=u2 > Threshold  Threshold=0.001  ZeroCross=off
  Switch1 : Switch  Criteria=u2 > Threshold  Threshold=0.001
  To Workspace1 : ToWorkspace  VariableName=Eta  SampleTime=[24 0]
  a4 : Constant
  eta : Outport
  tag scope: Irr=global
  wires:
  Add1/1 -> Divide/2, Scope4/1, Display3/1, Divide1/1
  [a1] -> Display2/1, Divide/3
  Divide1/1 -> Saturation1/1, Math Function/1
  [a2] -> Product/1, Display1/1
  Math Function/1 -> Product/2
  [Eta0] -> Add/1, Display/1
  Divide/1 -> Add/2, Scope2/1
  Product/1 -> Add/3
  Saturation/1 -> eta/1, Display4/1, Scope1/1, To Workspace1/1
  T ext/1 -> Add1/2
  Ti,coll/1 -> Add1/1
  H/1 -> Scope6/1, Switch/1, Switch/2, Switch1/2, Scope5/1, [Irr]
  Switch/1 -> Divide/1, Scope3/1, Display5/1, Product/3, Divide1/2
  Add/1 -> Switch1/1
  Constant/1 -> Switch1/3
  Switch1/1 -> Saturation/1
  Saturation1/1 -> Scope/1, Ascissa Climatica1/1
  a4/1 -> Switch/3

== system Model_HVAC_old_controller/Collector/Integral Block ==
  Watt : Inport
  Integrator : Integrator
  J to MJ : Gain  Gain=1/1000000
  MJ to kWh : Gain  Gain=1/3.6
  MJ1 : Display
  Scope1 : Scope
  Scope2 : Scope
  kWh1 : Display
  MJ : Outport  VectorParamsAs1DForOutWhenUnconnected=off
  kWh : Outport  Port=2  VectorParamsAs1DForOutWhenUnconnected=off
  wires:
  Integrator/1 -> J to MJ/1
  Watt/1 -> Integrator/1
  J to MJ/1 -> Scope1/1, MJ1/1, MJ/1, MJ to kWh/1
  MJ to kWh/1 -> Scope2/1, kWh1/1, kWh/1

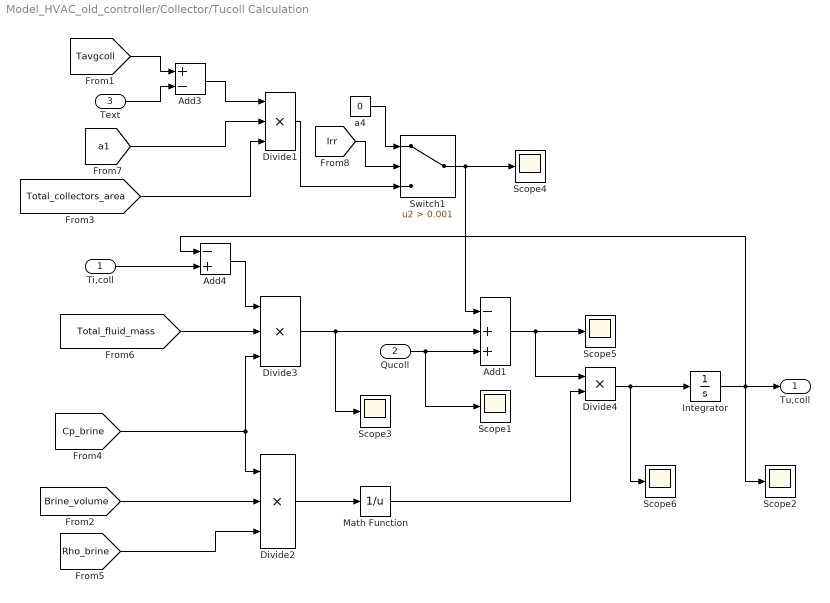
== system Model_HVAC_old_controller/Collector/Tucoll Calculation ==
  Ti,coll : Inport
  Qucoll : Inport  Port=2
  Text : Inport  Port=3
  Add1 : Sum  Inputs=-++
  Add3 : Sum  Inputs=+-
  Add4 : Sum  Inputs=-+
  Divide1 : Product  Inputs=***
  Divide2 : Product  Inputs=***
  Divide3 : Product  Inputs=***
  Divide4 : Product  Inputs=**
  Integrator : Integrator  InitialCondition=15
  Math Function : Math  Operator=reciprocal  SaturateOnIntegerOverflow=on
  Scope{1..6} (6 alike) : Scope
  Switch1 : Switch  Criteria=u2 > Threshold  Threshold=0.001
  a4 : Constant  Value=0
  Tu,coll : Outport  VectorParamsAs1DForOutWhenUnconnected=off
  wires:
  [Tavgcoll] -> Add3/1
  Text/1 -> Add3/2
  Add3/1 -> Divide1/1
  [a1] -> Divide1/2
  [Cp_brine] -> Divide2/1, Divide3/3
  [Brine_volume] -> Divide2/2
  [Rho_brine] -> Divide2/3
  Divide2/1 -> Math Function/1
  Ti,coll/1 -> Add4/2
  Divide1/1 -> Switch1/3
  Add4/1 -> Divide3/1
  Divide3/1 -> Add1/2, Scope3/1
  Qucoll/1 -> Add1/3, Scope1/1
  Add1/1 -> Divide4/1, Scope5/1
  Math Function/1 -> Divide4/2
  Divide4/1 -> Integrator/1, Scope6/1
  Integrator/1 -> Tu,coll/1, Scope2/1, Add4/1
  [Total_fluid_mass] -> Divide3/2
  [Total_collectors_area] -> Divide1/3
  [Irr] -> Switch1/2
  a4/1 -> Switch1/1
  Switch1/1 -> Add1/1, Scope4/1

== system Model_HVAC_old_controller/Collector/Utility ==
  Add4 : Sum
  Divide1 : Product  Inputs=**
  Divide5 : Product  Inputs=***
  Gain1 : Gain  Gain=1/2  SaturateOnIntegerOverflow=on  OutDataTypeStr=Inherit: Same as input  ParamDataTypeStr=Inherit: Same as input
  Product1 : Product  Inputs=**/  RndMeth=Zero
  contenuto1 : Constant  Value=1000
  tag scope: Brine_volume=global, Tavgcoll=global, Total_collectors_area=global, Total_fluid_mass=global
  wires:
  [Nc] -> Product1/1
  [L] -> Product1/2
  contenuto1/1 -> Product1/3
  Product1/1 -> [Brine_volume]
  [Aap] -> Divide5/3
  [Nc] -> Divide5/2
  [m_brine] -> Divide5/1
  Divide5/1 -> [Total_fluid_mass]
  [Aap] -> Divide1/2
  Divide1/1 -> [Total_collectors_area]
  [Nc] -> Divide1/1
  [Ticoll] -> Add4/1
  [Tucoll] -> Add4/2
  Add4/1 -> Gain1/1
  Gain1/1 -> [Tavgcoll]

== system Model_HVAC_old_controller/Pump/Integral Block ==
  Watt : Inport
  Integrator : Integrator
  J to MJ : Gain  Gain=1/1000000
  MJ to kWh : Gain  Gain=1/3.6
  MJ1 : Display
  Scope1 : Scope
  Scope2 : Scope
  kWh1 : Display
  MJ : Outport  VectorParamsAs1DForOutWhenUnconnected=off
  kWh : Outport  Port=2  VectorParamsAs1DForOutWhenUnconnected=off
  wires:
  Integrator/1 -> J to MJ/1
  Watt/1 -> Integrator/1
  J to MJ/1 -> Scope1/1, MJ1/1, MJ/1, MJ to kWh/1
  MJ to kWh/1 -> Scope2/1, kWh1/1, kWh/1

== system Model_HVAC_old_controller/Pump/Security System ==
  Tu,pump1 : Inport
  Tu,coll1 : Inport  Port=2
  Add2 : Sum  Inputs=+-
  Add3 : Sum  Inputs=+-
  Relay : Relay  OnSwitchValue=0  OffSwitchValue=-5  OnOutputValue=0  OffOutputValue=1
  Switch : Switch  Criteria=u2 > Threshold  ZeroCross=off
  Switch1 : Switch  Threshold=0.01  ZeroCross=off
  Switch2 : Switch  ZeroCross=off
  Tu,pump : Outport  VectorParamsAs1DForOutWhenUnconnected=off
  wires:
  Tu,coll1/1 -> Switch/3, Switch1/3, Switch2/3
  Tu,pump1/1 -> Switch/1
  Switch/1 -> Switch1/1
  [H] -> Switch1/2
  Switch1/1 -> Switch2/1, Add2/1
  Add2/1 -> Switch2/2
  Switch2/1 -> Tu,pump/1
  [T_s_max] -> Add3/2
  [T3] -> Add3/1, Add2/2
  Add3/1 -> Relay/1
  Relay/1 -> Switch/2

== system Model_HVAC_old_controller/Pump/Security System1 ==
  Pump power1 : Inport
  Add1 : Sum  Inputs=+-
  Add2 : Sum  Inputs=+-
  Constant : Constant  Value=0
  Relay : Relay  OnSwitchValue=0  OffSwitchValue=-5  OnOutputValue=0  OffOutputValue=1
  Scope1 : Scope
  Switch : Switch  Criteria=u2 > Threshold  ZeroCross=off
  Switch1 : Switch  Threshold=0.01  ZeroCross=off
  Pump power : Outport  VectorParamsAs1DForOutWhenUnconnected=off
  wires:
  Constant/1 -> Switch/3, Switch1/3
  [T_s_max] -> Add1/1
  [T3] -> Add1/2
  Pump power1/1 -> Switch/1
  [H] -> Switch1/2
  Switch/1 -> Switch1/1
  Switch1/1 -> Pump power/1
  [T_s_max] -> Add2/2
  [T3] -> Add2/1
  Add2/1 -> Relay/1
  Relay/1 -> Switch/2, Scope1/1

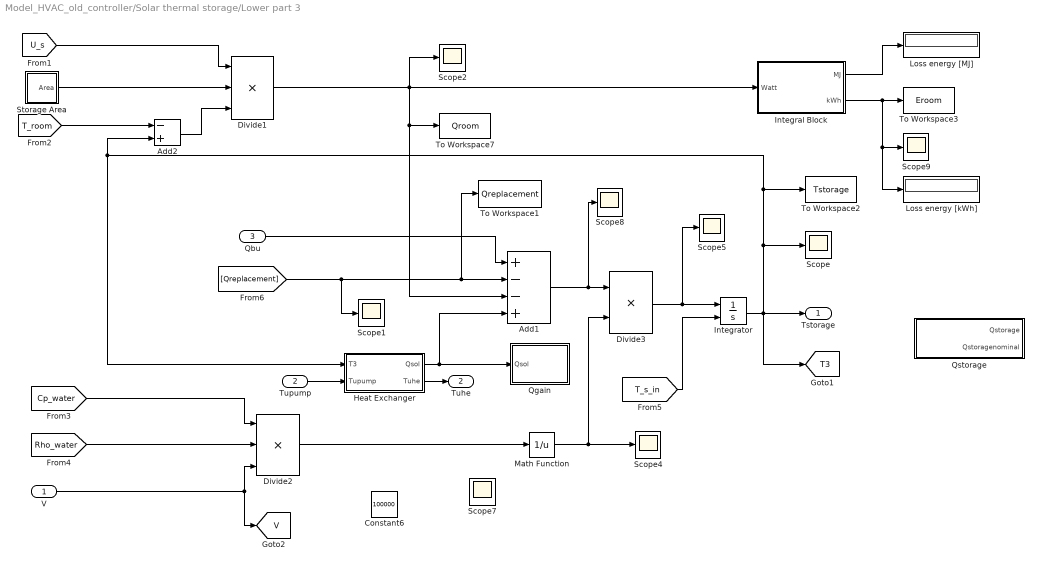
== system Model_HVAC_old_controller/Solar thermal storage/Lower part 3 ==
  V : Inport
  Tupump : Inport  Port=2
  Qbu : Inport  Port=3
  Add1 : Sum  Inputs=+--+
  Add2 : Sum  Inputs=-+
  Constant6 : Constant  Value=100000
  Divide1 : Product  Inputs=***
  Divide2 : Product  Inputs=***
  Divide3 : Product  Inputs=**
  Heat Exchanger : Subsystem
  Integral Block : Subsystem
  Integrator : Integrator  InitialConditionSource=external  InitialCondition=T_s_in
  Loss energy [MJ] : Display
      settings: Format=bank
  Loss energy [kWh] : Display
  Math Function : Math  Operator=reciprocal  SaturateOnIntegerOverflow=on
  Qgain : Subsystem
  Qstorage : Subsystem
  Scope{,1..2,4..5,7..9} (8 alike) : Scope
  Storage Area : Subsystem
  To Workspace1 : ToWorkspace  VariableName=Qreplacement  SampleTime=[24 0]
  To Workspace2 : ToWorkspace  VariableName=Tstorage  SampleTime=[24 0]
  To Workspace3 : ToWorkspace  VariableName=Eroom  SampleTime=[24 0]
  To Workspace7 : ToWorkspace  VariableName=Qroom  SampleTime=[24 0]
  Tstorage : Outport  VectorParamsAs1DForOutWhenUnconnected=off
  Tuhe : Outport  Port=2  VectorParamsAs1DForOutWhenUnconnected=off
  tag scope: T3=global, V=global
  wires:
  [Cp_water] -> Divide2/1
  [U_s] -> Divide1/1
  V/1 -> Divide2/3, [V]
  Divide1/1 -> To Workspace7/1, Add1/3, Integral Block/1(Watt), Scope2/1
  Divide2/1 -> Math Function/1
  Add1/1 -> Divide3/1, Scope8/1
  Math Function/1 -> Divide3/2, Scope4/1
  Divide3/1 -> Integrator/1, Scope5/1
  Integrator/1 -> [T3], Tstorage/1, Heat Exchanger/1(T3), Add2/2, To Workspace2/1, Scope/1
  [Rho_water] -> Divide2/2
  Heat Exchanger/1(Qsol) -> Add1/4, Qgain/1(Qsol)
  [T_room] -> Add2/1
  Heat Exchanger/2(Tuhe) -> Tuhe/1
  Add2/1 -> Divide1/3
  Storage Area/1(Area) -> Divide1/2
  [Qreplacement] -> Scope1/1, To Workspace1/1, Add1/2
  Tupump/1 -> Heat Exchanger/2(Tupump)
  Qbu/1 -> Add1/1
  Integral Block/1(MJ) -> Loss energy [MJ]/1
  Integral Block/2(kWh) -> To Workspace3/1, Scope9/1, Loss energy [kWh]/1
  [T_s_in] -> Integrator/2

== system Model_HVAC_old_controller/Back-up/Prova back-up/Controller Qbu ==
  If : If  NumInputs=2  IfExpression=u1>=u2  ZeroCross=off
  If Action Subsystem : Subsystem  TreatAsAtomicUnit=on
  If Action Subsystem3 : Subsystem  TreatAsAtomicUnit=on
  Merge : Merge
  Qbu : Outport  VectorParamsAs1DForOutWhenUnconnected=off
  wires:
  If/1 -> If Action Subsystem/Action
  If Action Subsystem/1(Out1) -> Merge/1
  Merge/1 -> Qbu/1
  If Action Subsystem3/1(Out1) -> Merge/2
  If/2 -> If Action Subsystem3/Action
  [Qstorage] -> If/1
  [Qstoragenominal] -> If/2
  [BU_power] -> If Action Subsystem3/1(In1)

== system Model_HVAC_old_controller/Back-up/Prova back-up/Qstored ==
  Add2 : Sum  Inputs=-+
  Product3 : Product  Inputs=***  SaturateOnIntegerOverflow=on  OutDataTypeStr=Inherit: Same as first input
  Qstored : Outport  VectorParamsAs1DForOutWhenUnconnected=off
  wires:
  Product3/1 -> Qstored/1
  [Tacq] -> Add2/1
  [T3] -> Add2/2
  Add2/1 -> Product3/1
  [m] -> Product3/2
  [Cp_water] -> Product3/3

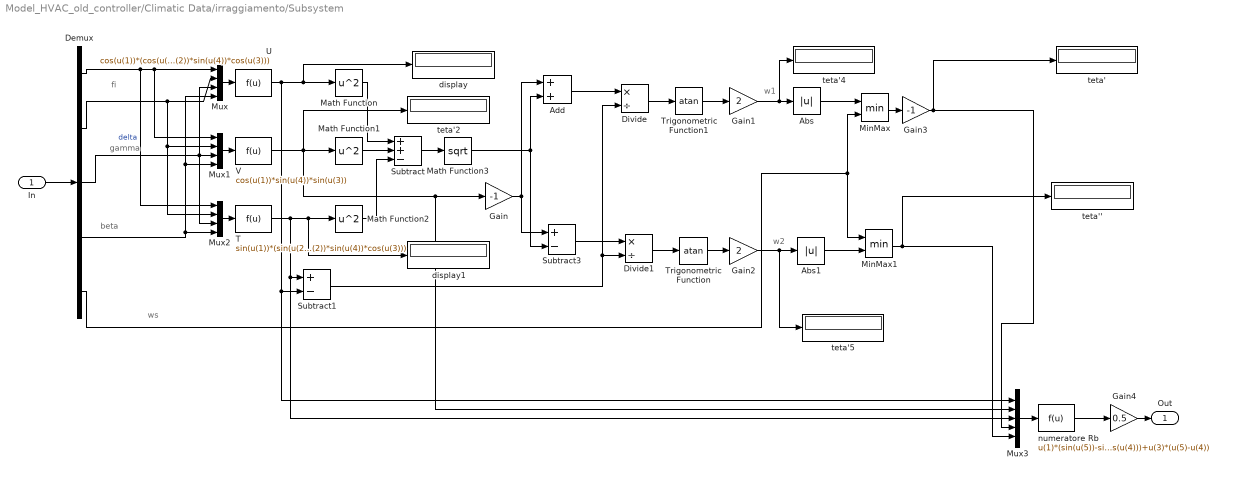
== system Model_HVAC_old_controller/Climatic Data/irraggiamento/Subsystem ==
  note: w1
  note: w2
  note: fi
  note: ws
  note: gamma
  note: beta
  In : Inport
  Abs : Abs
  Abs1 : Abs
  Add : Sum
  Demux : Demux  Outputs=5
  Divide : Product  Inputs=*/
  Divide1 : Product  Inputs=*/
  Gain : Gain  Gain=-1
  Gain1 : Gain  Gain=2
  Gain2 : Gain  Gain=2
  Gain3 : Gain  Gain=-1
  Gain4 : Gain  Gain=0.5
  Math Function : Math  Operator=square  SaturateOnIntegerOverflow=on
  Math Function1 : Math  Operator=square  SaturateOnIntegerOverflow=on
  Math Function2 : Math  Operator=square  SaturateOnIntegerOverflow=on
  Math Function3 : Math  Operator=sqrt  SaturateOnIntegerOverflow=on
  MinMax : MinMax  Inputs=2
  MinMax1 : MinMax  Inputs=2
  Mux : Mux
  Mux1 : Mux
  Mux2 : Mux
  Mux3 : Mux  Inputs=5
  Subtract : Sum  Inputs=++-
  Subtract1 : Sum  Inputs=+-
  Subtract3 : Sum  Inputs=+-
  T : Fcn  Expr=sin(u(1))*(sin(u(2))*cos(u(4))-cos(u(2))*sin(u(4))*cos(u(3)))
  Trigonometric Function : Trigonometry  Operator=atan
  Trigonometric Function1 : Trigonometry  Operator=atan
  U : Fcn  Expr=cos(u(1))*(cos(u(2))*cos(u(4))+sin(u(2))*sin(u(4))*cos(u(3)))
  V : Fcn  Expr=cos(u(1))*sin(u(4))*sin(u(3))
  display : Display
  display1 : Display
  numeratore Rb : Fcn  Expr=u(1)*(sin(u(5))-sin(u(4)))-u(2)*(cos(u(5))-cos(u(4)))+u(3)*(u(5)-u(4))
  teta'{,2,4..5} (4 alike) : Display
  teta'' : Display
  Out : Outport  VectorParamsAs1DForOutWhenUnconnected=off
  wires:
  Mux1/1 -> V/1
  Mux/1 -> U/1
  Mux2/1 -> T/1
  Demux/1 -> Mux/1, Mux1/1, Mux2/1  "delta"
  Demux/2 -> Mux/2, Mux1/2, Mux2/2
  T/1 -> Subtract1/1, Mux3/3, Math Function2/1, display1/1
  V/1 -> Math Function1/1, Gain/1, Mux3/2, teta'2/1
  U/1 -> Subtract1/2, Mux3/1, Math Function/1, display/1
  Math Function2/1 -> Subtract/3
  Math Function1/1 -> Subtract/2
  Math Function/1 -> Subtract/1
  Subtract/1 -> Math Function3/1
  Gain/1 -> Subtract3/1, Add/1
  Math Function3/1 -> Add/2, Subtract3/2
  Add/1 -> Divide/1
  Subtract3/1 -> Divide1/1
  Subtract1/1 -> Divide1/2, Divide/2
  Divide/1 -> Trigonometric Function1/1
  Divide1/1 -> Trigonometric Function/1
  Trigonometric Function1/1 -> Gain1/1
  Trigonometric Function/1 -> Gain2/1
  Gain2/1 -> Abs1/1, teta'5/1
  Gain1/1 -> Abs/1, teta'4/1
  Abs/1 -> MinMax/1
  MinMax/1 -> Gain3/1
  Demux/5 -> MinMax/2, MinMax1/1
  Abs1/1 -> MinMax1/2
  Gain3/1 -> teta'/1, Mux3/4
  MinMax1/1 -> teta''/1, Mux3/5
  Mux3/1 -> numeratore Rb/1
  numeratore Rb/1 -> Gain4/1
  Gain4/1 -> Out/1
  In/1 -> Demux/1
  Demux/3 -> Mux/3, Mux1/3, Mux2/3
  Demux/4 -> Mux/4, Mux1/4, Mux2/4

== system Model_HVAC_old_controller/Climatic Data/irraggiamento/ws1 ==
  Delta : Inport
  Phi : Inport  Port=2
  Mux1 : Mux  Inputs=2
  Sum : Sum  Inputs=|-+  SaturateOnIntegerOverflow=on
  alba : Display
  cosws : Fcn  Expr=-tan(u[1])*tan(u[2])
  kWh annue2 : Display
  rad grad1 : Fcn  Expr=12-u[1]/15
  rad grad2 : Fcn  Expr=u[1]/pi*180
  rad grad3 : Fcn  Expr=12+u[1]/15
  tramonto : Display
  wsx : Trigonometry  Operator=acos
  Day Length : Outport  VectorParamsAs1DForOutWhenUnconnected=off
  ws : Outport  Port=2  VectorParamsAs1DForOutWhenUnconnected=off
  wires:
  Phi/1 -> Mux1/2
  Delta/1 -> Mux1/1
  rad grad2/1 -> rad grad3/1, rad grad1/1, kWh annue2/1
  wsx/1 -> rad grad2/1, ws/1
  cosws/1 -> wsx/1
  Mux1/1 -> cosws/1
  rad grad1/1 -> alba/1, Sum/1
  rad grad3/1 -> tramonto/1, Sum/2
  Sum/1 -> Day Length/1

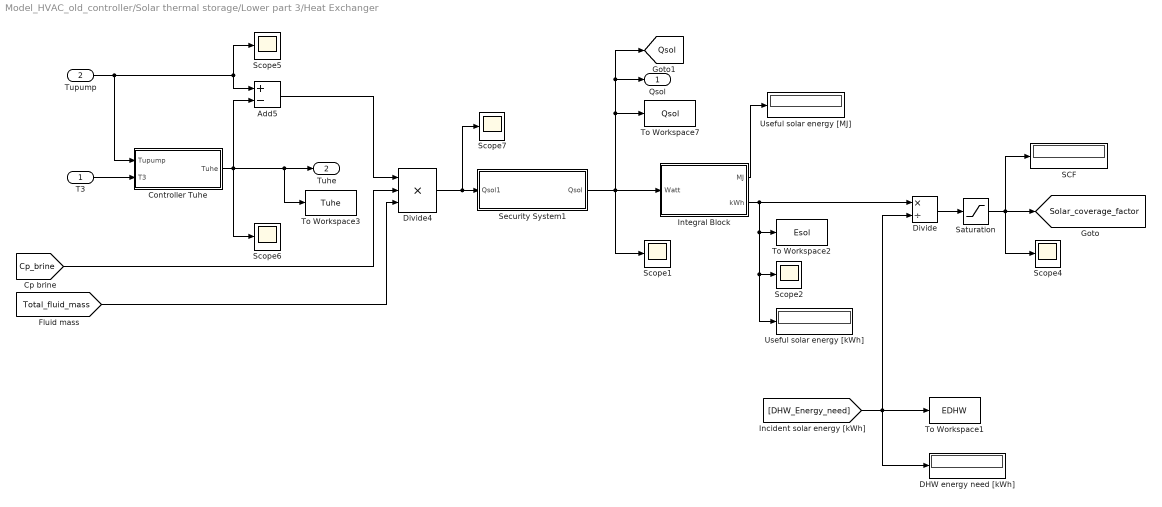
== system Model_HVAC_old_controller/Solar thermal storage/Lower part 3/Heat Exchanger ==
  T3 : Inport
  Tupump : Inport  Port=2
  Add5 : Sum  Inputs=+-
  Controller Tuhe : Subsystem
  DHW energy need [kWh] : Display
  Divide : Product  Inputs=*/
  Divide4 : Product  Inputs=***
  Integral Block : Subsystem
  SCF : Display
  Saturation : Saturate  UpperLimit=1  LowerLimit=0
  Scope{1..2,4..7} (6 alike) : Scope
  Security System1 : Subsystem
  To Workspace1 : ToWorkspace  VariableName=EDHW  SampleTime=[24 0]
  To Workspace2 : ToWorkspace  VariableName=Esol  SampleTime=[24 0]
  To Workspace3 : ToWorkspace  VariableName=Tuhe  SampleTime=[24 0]
  To Workspace7 : ToWorkspace  VariableName=Qsol  SampleTime=[24 0]
  Useful solar energy [MJ] : Display
      settings: Format=bank
  Useful solar energy [kWh] : Display
  Qsol : Outport  VectorParamsAs1DForOutWhenUnconnected=off
  Tuhe : Outport  Port=2  VectorParamsAs1DForOutWhenUnconnected=off
  tag scope: Qsol=global, Solar_coverage_factor=global
  wires:
  Tupump/1 -> Add5/1, Scope5/1, Controller Tuhe/1(Tupump)
  Add5/1 -> Divide4/1
  [Cp_brine] -> Divide4/2
  [Total_fluid_mass] -> Divide4/3
  Divide/1 -> Saturation/1
  Saturation/1 -> Scope4/1, SCF/1, [Solar_coverage_factor]
  Security System1/1(Qsol) -> Integral Block/1(Watt), To Workspace7/1, Qsol/1, [Qsol], Scope1/1
  Divide4/1 -> Security System1/1(Qsol1), Scope7/1
  T3/1 -> Controller Tuhe/2(T3)
  Controller Tuhe/1(Tuhe) -> Add5/2, Scope6/1, Tuhe/1, To Workspace3/1
  Integral Block/1(MJ) -> Useful solar energy [MJ]/1
  Integral Block/2(kWh) -> Divide/1, To Workspace2/1, Scope2/1, Useful solar energy [kWh]/1
  [DHW_Energy_need] -> Divide/2, To Workspace1/1, DHW energy need [kWh]/1

== system Model_HVAC_old_controller/Solar thermal storage/Lower part 3/Integral Block ==
  Watt : Inport
  Integrator : Integrator
  J to MJ : Gain  Gain=1/1000000
  MJ to kWh : Gain  Gain=1/3.6
  MJ1 : Display
  Scope1 : Scope
  Scope2 : Scope
  kWh1 : Display
  MJ : Outport  VectorParamsAs1DForOutWhenUnconnected=off
  kWh : Outport  Port=2  VectorParamsAs1DForOutWhenUnconnected=off
  wires:
  Integrator/1 -> J to MJ/1
  Watt/1 -> Integrator/1
  J to MJ/1 -> Scope1/1, MJ1/1, MJ/1, MJ to kWh/1
  MJ to kWh/1 -> Scope2/1, kWh1/1, kWh/1

== system Model_HVAC_old_controller/Solar thermal storage/Lower part 3/Qgain ==
  Qsol : Inport
  Controller Qgain : Subsystem
  DHW energy need [kWh] : Display
  Divide : Product  Inputs=/*
  Gained energy [MJ] : Display
      settings: Format=bank
  Gained energy [kWh] : Display
  Integral Block : Subsystem
  SCF : Display
  Saturation : Saturate  UpperLimit=1  LowerLimit=0
  Scope1 : Scope
  Scope4 : Scope
  Scope5 : Scope
  To Workspace1 : ToWorkspace  VariableName=Qgain  SampleTime=[24 0]
  To Workspace3 : ToWorkspace  VariableName=Egain  SampleTime=[24 0]
  wires:
  Divide/1 -> Saturation/1
  Saturation/1 -> Scope4/1, SCF/1
  [DHW_Energy_need] -> Divide/1, DHW energy need [kWh]/1
  [Qwhr] -> Controller Qgain/1(Qwhr)
  Controller Qgain/1(Qgain) -> To Workspace1/1, Scope1/1, Integral Block/1(Watt)
  Integral Block/1(MJ) -> Gained energy [MJ]/1
  Integral Block/2(kWh) -> Divide/2, To Workspace3/1, Scope5/1, Gained energy [kWh]/1
  Qsol/1 -> Controller Qgain/2(Qsol)

== system Model_HVAC_old_controller/Solar thermal storage/Lower part 3/Qstorage ==
  Add1 : Sum  Inputs=-+
  Add2 : Sum  Inputs=-+
  Gain : Gain  Gain=1/3600
  Gain1 : Gain  Gain=1/3600
  Gained energy [kWh]1 : Display
  Gained energy [kWh]2 : Display
  Product1 : Product  Inputs=****  SaturateOnIntegerOverflow=on  OutDataTypeStr=Inherit: Same as first input
  Product3 : Product  Inputs=****  SaturateOnIntegerOverflow=on  OutDataTypeStr=Inherit: Same as first input
  Scope1 : Scope
  Scope2 : Scope
  Qstorage : Outport  VectorParamsAs1DForOutWhenUnconnected=off
  Qstoragenominal : Outport  Port=2  VectorParamsAs1DForOutWhenUnconnected=off
  tag scope: Qstorage=global, Qstoragenominal=global
  wires:
  [T_acq] -> Add2/1
  [T3] -> Add2/2
  Add2/1 -> Product3/1
  [Rho_water] -> Product3/2
  [Cp_water] -> Product3/3
  [V] -> Product3/4
  Product3/1 -> Gain/1
  Gain/1 -> Qstorage/1, Scope1/1, Gained energy [kWh]1/1, [Qstorage]
  [T_acq] -> Add1/1
  [T_DHW] -> Add1/2
  Add1/1 -> Product1/1
  [Rho_water] -> Product1/2
  [Cp_water] -> Product1/3
  [V] -> Product1/4
  Product1/1 -> Gain1/1
  Gain1/1 -> Qstoragenominal/1, Scope2/1, Gained energy [kWh]2/1, [Qstoragenominal]
